simulink model "serial_communication"  (R2020a)
settings: Solver=FixedStepAuto  StartTime=0.0  StopTime=10.0  FixedStep=1e-3  RelTol=1e-3  EnableMultiTasking=on
libraries: frdmk64flib x5, etargetslib x2
settings Model: ExtModeTrigDuration=5  Creator=Ethan  LastModifiedBy=Ethan
settings OptimizationCC: EnhancedBackFolding=on  PassReuseOutputArgsAs=Individual arguments  ZeroExternalMemoryAtStartup=off  ZeroInternalMemoryAtStartup=off  MaxStackSize=64  OptimizeBlockOrder=speed  DifferentSizesBufferReuse=on  OptimizationCustomize=off  EfficientTunableParamExpr=on
settings DebuggingCC: ParameterTunabilityLossMsg=error
settings HardwareCC: ProdBitPerPointer=32  ProdBitPerSizeT=32  ProdBitPerPtrDiffT=32  ProdLargestAtomicInteger=Long  ProdLargestAtomicFloat=Double  ProdWordSize=32  ProdHWDeviceType=ARM Compatible->ARM Cortex
settings SFSimCC: MATLABDynamicMemAlloc=off
settings RTWCC: SystemTargetFile=ert.tlc  HardwareBoard=NXP FRDM-K64F  TemplateMakefile=ert_default_tmf  Toolchain=GNU Tools for ARM Embedded Processors
settings CodeAppCC: ForceParamTrailComments=on  IgnoreCustomStorageClasses=off  OperatorAnnotations=on  SimulinkDataObjDesc=on  SFDataObjDesc=on  InsertBlockDesc=on

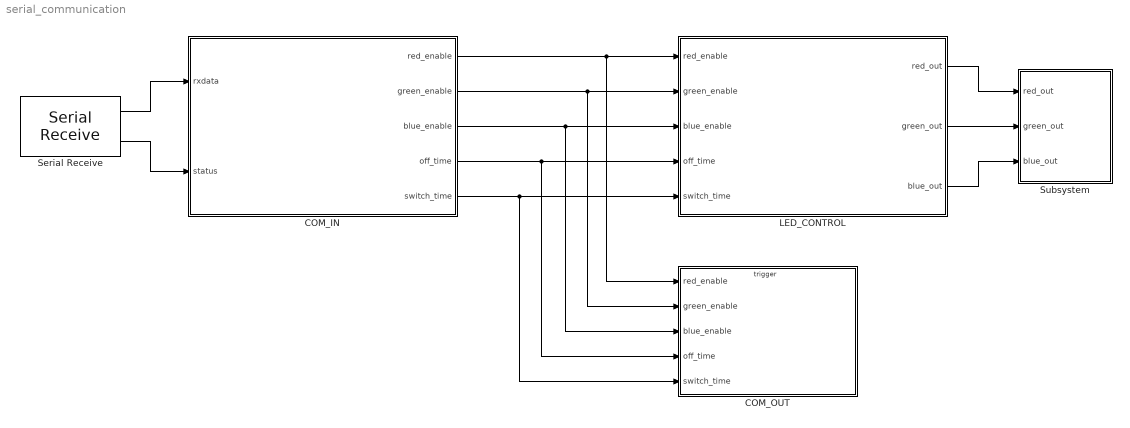
== system serial_communication ==
  COM_IN : Stateflow chart  TreatAsAtomicUnit=on
      settings: PortSchema="{\"entries\":[{\"content\":{\"sides\":[{\"content\":{\"connectorIds\":[\"In1\",\"In2\"]},\"type\":\"ConnectorPlacement.EquallySpacedRectSide\",\"uuid\":\"483f875f-8122-4417-a61a-7c7c36b8fce3\"},{\"content\":{\"connectorIds\":[\"Out3\",\"Out4\",\"Out5\",\"Out1\",\"Out2\"],\"side\":\"RIGHT\"},\"type\":\"ConnectorPlacement.EquallySpacedRectSide\",\"uuid\":\"d5d74415-f253-4c25-91ca-72d167cc5f74\"},{\"content\":{\"connectorIds\":[],\"side\":\"TOP\"},\"type\":\"ConnectorPlacement.EquallySpacedRectSide\",\"uuid\":\"3ac4d4af-1043-40bc-bae2-faa226735a1b\"}]},\"type\":\"ConnectorPlacement.EquallySpacedConnector\",\"uuid\":\"0e01a1ca-0d7b-47c5-ac0f-4eceb0548e92\"}],\"packageUris\":[\"http://schema.mathworks.com/mf0/Connector/19700101\"],\"version\":\"1.0\"}"
  COM_OUT : Subsystem
  LED_CONTROL : Stateflow chart  TreatAsAtomicUnit=on
      settings: PortSchema="{\"entries\":[{\"content\":{\"sides\":[{\"content\":{\"connectorIds\":[\"In4\",\"In2\",\"In1\",\"In3\",\"In5\"]},\"type\":\"ConnectorPlacement.EquallySpacedRectSide\",\"uuid\":\"8e3ecd85-9bff-4d68-8ffe-d0e8e8a3e875\"},{\"content\":{\"connectorIds\":[\"Out3\",\"Out2\",\"Out1\"],\"side\":\"RIGHT\"},\"type\":\"ConnectorPlacement.EquallySpacedRectSide\",\"uuid\":\"0f3495a6-79b1-4f5a-8162-7ca1b8857a43\"},{\"content\":{\"connectorIds\":[],\"side\":\"TOP\"},\"type\":\"ConnectorPlacement.EquallySpacedRectSide\",\"uuid\":\"b7d7e845-f65f-4412-a13d-1fb698e23000\"}]},\"type\":\"ConnectorPlacement.EquallySpacedConnector\",\"uuid\":\"29845ac7-8384-4e32-baec-b5c431bbadf5\"}],\"packageUris\":[\"http://schema.mathworks.com/mf0/Connector/19700101\"],\"version\":\"1.0\"}"
  Serial Receive : frdmk64flib/Serial Receive  SCIModule=0  Baudrate=uint32(9600)  Parity=None  StopBits=1  HardwareFlowControl=None  ByteOrder=LittleEndian  DataType=uint8  DataLength=11  BlockingMode=off  OutputStatus=on  SampleTime=-1
  Subsystem : Subsystem
  wires:
  Serial Receive/1 -> COM_IN/1(rxdata)
  Serial Receive/2 -> COM_IN/2(status)
  COM_IN/3(red_enable) -> COM_OUT/1(red_enable), LED_CONTROL/4(red_enable)
  COM_IN/4(green_enable) -> COM_OUT/2(green_enable), LED_CONTROL/2(green_enable)
  COM_IN/5(blue_enable) -> COM_OUT/3(blue_enable), LED_CONTROL/1(blue_enable)
  COM_IN/1(off_time) -> LED_CONTROL/3(off_time), COM_OUT/4(off_time)
  COM_IN/2(switch_time) -> LED_CONTROL/5(switch_time), COM_OUT/5(switch_time)
  LED_CONTROL/3(red_out) -> Subsystem/1(red_out)
  LED_CONTROL/2(green_out) -> Subsystem/2(green_out)
  LED_CONTROL/1(blue_out) -> Subsystem/3(blue_out)

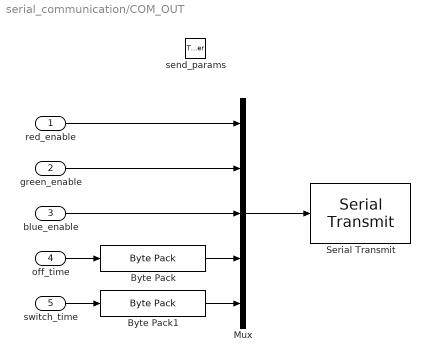
== system serial_communication/COM_OUT ==
  red_enable : Inport
  green_enable : Inport  Port=2
  blue_enable : Inport  Port=3
  off_time : Inport  Port=4
  switch_time : Inport  Port=5
  send_params : TriggerPort  TriggerType=function-call  IsSimulinkFunction=on  FunctionName=send_params  VariantControl=Variant
  Byte Pack : etargetslib/Byte Pack  datatypes={'single'}  byteAlign=1
  Byte Pack1 : etargetslib/Byte Pack  datatypes={'uint16'}  byteAlign=1
  Mux : Mux  Inputs=5
  Serial Transmit : frdmk64flib/Serial Transmit  SCIModule=0  Baudrate=uint32(9600)  Parity=None  StopBits=1  HardwareFlowControl=None  ByteOrder=LittleEndian  BlockingMode=on  OutputStatus=off
  wires:
  Byte Pack/1 -> Mux/4
  off_time/1 -> Byte Pack/1
  green_enable/1 -> Mux/2
  switch_time/1 -> Byte Pack1/1
  red_enable/1 -> Mux/1
  Mux/1 -> Serial Transmit/1
  blue_enable/1 -> Mux/3
  Byte Pack1/1 -> Mux/5

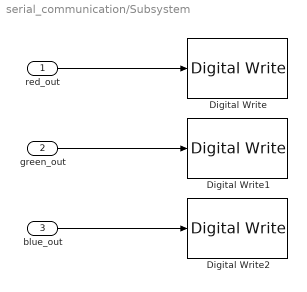
== system serial_communication/Subsystem ==
  red_out : Inport
  green_out : Inport  Port=2
  blue_out : Inport  Port=3
  Digital Write : frdmk64flib/Digital Write  Whichpin=RED_LED
  Digital Write1 : frdmk64flib/Digital Write  Whichpin=GREEN_LED
  Digital Write2 : frdmk64flib/Digital Write  Whichpin=BLUE_LED
  wires:
  blue_out/1 -> Digital Write2/1
  green_out/1 -> Digital Write1/1
  red_out/1 -> Digital Write/1

== stateflow chart serial_communication/LED_CONTROL ==
  state OFF
    entry:
    red_out = 0;
    green_out = 0;
    blue_out = 0;
  state RED_ON
    entry:
    red_out = 1;
    green_out = 0;
    blue_out = 0;
  state BLUE_ON
    entry:
    red_out = 0;
    green_out = 0;
    blue_out = 1;
  state GREEN_ON
    entry:
    red_out = 0;
    green_out = 1;
    blue_out = 0;
  (default) -> OFF
  OFF -> (junction 3) : after(off_time,sec)
  (junction 3) -> RED_ON [order 1] : [red_enable == 1]
  (junction 3) -> (junction 8) [order 2]
  (junction 7) -> OFF
  RED_ON -> (junction 8) : after(switch_time, msec)
  (junction 9) -> (junction 7) [order 2]
  (junction 8) -> (junction 9) [order 2]
  BLUE_ON -> (junction 7) : after(switch_time, msec)
  (junction 8) -> GREEN_ON [order 1] : [green_enable == 1]
  (junction 9) -> BLUE_ON [order 1] : [blue_enable == 1]
  GREEN_ON -> (junction 9) : after(switch_time, msec)
  data: blue_enable input; green_enable input; off_time input; red_enable input; blue_out output; green_out output; red_out output; switch_time input

== stateflow chart serial_communication/COM_IN ==
  settings: executeAtInitialization=1
  state SET_PARAM
    entry:
    red_enable =rxdata(3);
    green_enable = rxdata(4);
    blue_enable = rxdata(5);
    off_time = typecast(rxdata(6:9), 'single');
    switch_time = typecast(rxdata(10:11), 'uint16');
  state INITIAL
    entry:
    red_enable = 1;
    green_enable = 1;
    blue_enable = 0;
    off_time = 0.5; % in sec
    switch_time = 200; %in ms
  state STANDBY
    %waiting for com
  state ECHO_PARAM
    entry:
    send_params();
  SET_PARAM -> STANDBY
  (default) -> INITIAL
  (junction 11) -> SET_PARAM [order 1] : [rxdata(2) == hex2dec('55')]
  (junction 5) -> STANDBY [order 2]
  INITIAL -> STANDBY
  STANDBY -> (junction 5) : [status == 0]
  (junction 5) -> (junction 11) [order 1] : [rxdata(1) == hex2dec('16')]
  (junction 11) -> ECHO_PARAM [order 2] : [rxdata(2) == hex2dec('22')]
  ECHO_PARAM -> STANDBY
  data: rxdata input uint8; status input uint8; off_time output single; switch_time output uint16; red_enable output uint8; green_enable output uint8; blue_enable output uint8
